simulink model "nimbus"  (R2015b)
settings: Solver=FixedStepDiscrete  SolverMode=SingleTasking  StartTime=0.0  StopTime=sim_stop_time  FixedStep=sim_time_step_size  RelTol=1e-3
PreLoadFcn:
  | nimbus_bus_all;
values from neighbouring files (symbols this model uses):
  sim_time_step_size = 1/100    (= 0.01)    [nimbus_sim_init.m]
undefined symbols (not defined in the file or in its folder): accel, cam_cam1_lander_dcm, cam_cam1_lander_quat, cam_cam1_pos_in_lander, cam_processing_delay_cycles, central_body_flattening, central_body_radius, central_body_rotation_rate, csc_ekf_nonlinear_filter_lib, csc_ekf_nonlinear_filter_new, csc_est_state_est_new, csc_estimation_lib, csc_kfl_kalman_filter_lib, csc_kfl_kalman_filter_new, csc_ldr_flir_lidar, csc_ldr_flir_lidar_lib, csc_rsp_radar_sensor_prep_lib, csc_rsp_radar_sensor_prep_new, csc_sensors_a, csc_sensors_lib_a, csc_sim_simulation, csc_sim_simulation_lib, csc_snp_sensor_prep_lib, csc_snp_sensor_prep_new, csci_fsw, csci_fsw_lib, csci_gsse, csci_gsse_lib, est_time_step, fcv_initializing, ini_alt_wrt_meanrad, ini_epoch_seconds, kfl_lidar_switch_altitude, kfl_use_range_meas, ldr_lander_dcm, ldr_use_meme_flag, pwr_ldr_on_state, q, snp_dtheta_filter_coeffs, snp_dtheta_filter_order, snp_meas_noise_alt, snp_meas_noise_angle, snp_meas_noise_angle_exp, snp_meas_noise_angle_gain, snp_meas_noise_dtheta, snp_meas_noise_dtheta_exp, snp_meas_noise_dtheta_gain, snp_meas_noise_indep, snp_R_lower_limit_alt, snp_R_lower_limit_angle, snp_R_lower_limit_dtheta, snp_rdr_index, snp_rdr_zero_index, snp_zero_index, snp_zero_meas, swm_num_switches, x
undefined symbols (not defined in the file): ldr_position_in_lander
libraries: util_common_lib x23, util_info_lib x13, simulink x8, util_frame_rotation_lib x5, util_quat_lib x5, simulink_extras x4, util_geodesy_lib x2, csu_cfe_cfe_time_lib x2, csu_tlm_telemetry_lib x2, csu_flr_lidar_noise_model_lib x2, csc_act_actuator_manager_lib x1, csc_cmp_command_mode_process_lib x1
(part 1 of 2)
settings Model: SimulationMode=rapid-accelerator  ExtModeTrigDuration=100  Creator=ianmga  LastModifiedBy=Mark Agbayani
settings DataIOCC: LimitDataPoints=off  SaveFormat=Array  SaveOutput=off  SaveTime=off  StateSaveName=tmp_raccel_xout  SignalLoggingName=raw_event_logs
settings OptimizationCC: ExpressionDepthLimit=2147483647  InitFltsAndDblsToZero=on  OptimizeModelRefInitCode=on
settings DebuggingCC: CheckSSInitialOutputMsg=off  UnderspecifiedInitializationDetection=Classic  SolverPrmCheckMsg=warning  InheritedTsInSrcMsg=none  UnderSpecifiedDataTypeMsg=warning  FcnCallInpInsideContextMsg=UseLocalSettings  BusObjectLabelMismatch=error  StateNameClashWarn=warning  StrictBusMsg=WarnOnBusTreatedAsVector
settings HardwareCC: ProdBitPerPointer=32  ProdLargestAtomicFloat=None  ProdIntDivRoundTo=Undefined  ProdEndianess=Unspecified  ProdWordSize=32  ProdHWDeviceType=32-bit Generic  TargetHWDeviceType=32-bit Generic
settings SFSimCC: SimParseCustomCode=off
settings SFSimCC: SimUserIncludeDirs=|
  | sim/fhw/sensors/cameras/kir
  | fsw/est/kcv
  | fsw/est/kfd
  | externals/minopencv/include
settings RTWCC: SystemTargetFile=ert.tlc  GenCodeOnly=on  TemplateMakefile=ert_default_tmf  Description=Embedded Coder  RetainRTWFile=on  RTWUseSimCustomCode=on
settings RTWCC: CustomInclude=|
  | sim/fhw/sensors/cameras/kir
  | fsw/est/kcv
  | fsw/est/kfd
  | externals/minopencv/include
settings CodeAppCC: ForceParamTrailComments=on  IgnoreCustomStorageClasses=off  MaxIdLength=128  SimulinkDataObjDesc=on  SFDataObjDesc=on  MangleLength=10  CustomSymbolStrType=$N$R$M  InsertBlockDesc=on  InternalIdentifier=Classic  ReqsInCode=on
settings ERTTargetCC: GenerateSampleERTMain=on  MultiInstanceERTCode=on  CodeInterfacePackaging=Reusable function  RootIOFormat=Structure reference  ERTCustomFileTemplate=csl_interface.tlc
settings ConfigComp: CovModelRefEnable=Off  CovSFcnEnable=off

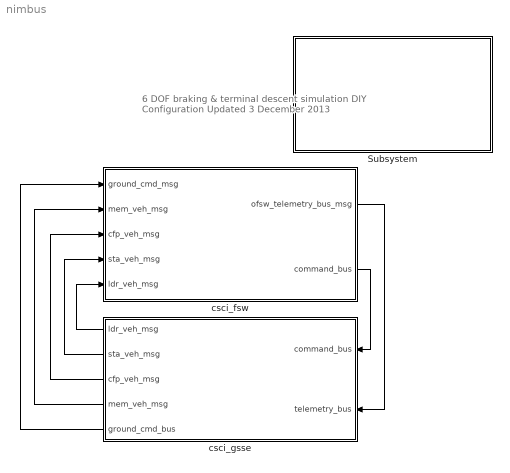
== system nimbus ==
  note: 6 DOF braking & terminal descent simulation
      | DIY Configuration
      |
      | Updated 3 December 2013
  Subsystem : Subsystem
      mask Display: image('nimbus.png')
  csci_fsw : Subsystem  AncestorBlock=csci_fsw_lib/csci_fsw
  csci_gsse : Subsystem  AncestorBlock=csci_gsse_lib/csci_gsse
  wires:
  csci_fsw/2(command_bus) -> csci_gsse/1(command_bus)
  csci_fsw/1(ofsw_telemetry_bus_msg) -> csci_gsse/2(telemetry_bus)
  csci_gsse/1(ldr_veh_msg) -> csci_fsw/5(ldr_veh_msg)
  csci_gsse/2(sta_veh_msg) -> csci_fsw/4(sta_veh_msg)
  csci_gsse/3(cfp_veh_msg) -> csci_fsw/3(cfp_veh_msg)
  csci_gsse/5(ground_cmd_bus) -> csci_fsw/1(ground_cmd_msg)
  csci_gsse/4(mem_veh_msg) -> csci_fsw/2(mem_veh_msg)

== system nimbus/Subsystem ==

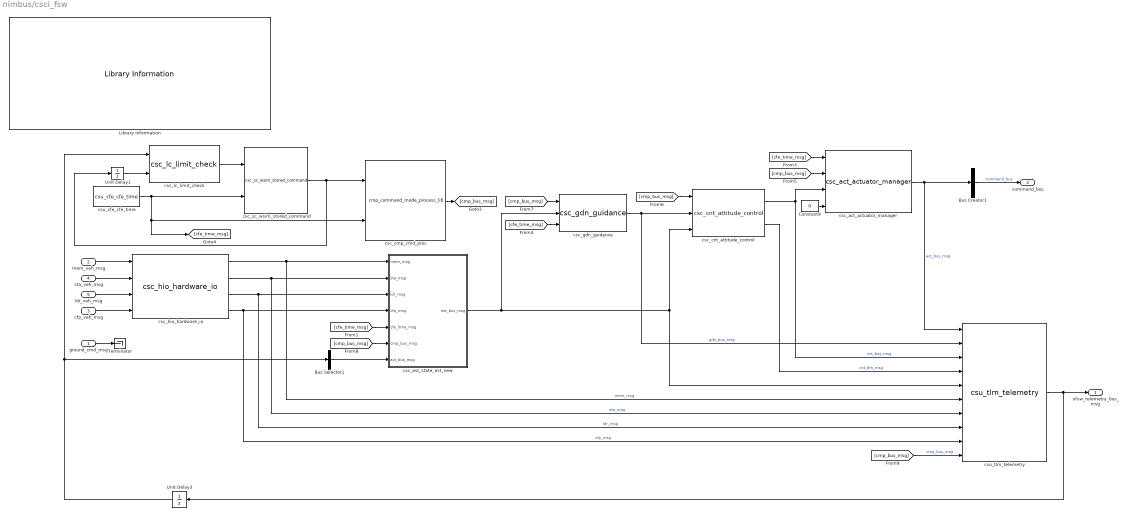
== system nimbus/csci_fsw ==
  ground_cmd_msg : Inport
  mem_veh_msg : Inport  Port=2
  cfp_veh_msg : Inport  Port=3
  sta_veh_msg : Inport  Port=4
  ldr_veh_msg : Inport  Port=5
  Bus Creator1 : BusCreator  Inputs=1
  Bus Selector1 : BusSelector  OutputSignals=act_bus_msg  OutputAsBus=on
  Constant9 : Constant  Value=0  OutDataTypeStr=uint32
  Library Information : util_info_lib/Library Information  owner='NONE'
  Terminator : Terminator
  Unit Delay1 : UnitDelay  SampleTime=-1
  Unit Delay3 : UnitDelay  SampleTime=-1
  csc_act_actuator_manager : csc_act_actuator_manager_lib/csc_act_actuator_manager  Tag=OFSW; MDL_TICK=CNT_BUS_MSG
  csc_cmp_cmd_proc : csc_cmp_command_mode_process_lib/cmp_command_mode_process_lib  Tag=OFSW
  csc_cnt_attitude_control : csc_cnt_attitude_control_lib/csc_cnt_attitude_control  Tag=OFSW; MDL_TICK=GDN_BUS_MSG
  csc_est_state_est_new : Subsystem  Tag=OFSW; MDL_TICK=CMP_BUS_MSG  AncestorBlock=csc_estimation_lib/csc_est_state_est_new  TreatAsAtomicUnit=on  SystemSampleTime=est_time_step
  csc_gdn_guidance : csc_gdn_guidance_lib/csc_gdn_guidance  Tag=OFSW; MDL_TICK=EST_BUS_MSG
  csc_hio_hardware_io : csc_hio_hardware_io_lib/csc_hio_hardware_io
  csc_lc_limit_check : csc_lc_limit_check_lib/csc_lc_limit_check
  csc_sc_wsim_stored_command : csc_sc_wsim_stored_command_lib/csc_sc_wsim_stored_command
  csu_cfe_cfe_time : csu_cfe_cfe_time_lib/csu_cfe_cfe_time  sch_dt=fsw_dt
  csu_tlm_telemetry : csu_tlm_telemetry_lib/csu_tlm_telemetry  num_inputs=10  output_bus_name=ofsw_telemetry_bus_msg
  ofsw_telemetry_bus_msg : Outport
  command_bus : Outport  Port=2
  wires:
  Unit Delay1/1 -> csc_lc_limit_check/2
  Unit Delay3/1 -> csc_lc_limit_check/1, Bus Selector1/1
  csc_lc_limit_check/1 -> csc_sc_wsim_stored_command/1
  [cmp_bus_msg] -> csu_tlm_telemetry/10  "cmp_bus_msg"
  csc_hio_hardware_io/4 -> csc_est_state_est_new/4(cfp_msg), csu_tlm_telemetry/9  "cfp_msg"
  csc_hio_hardware_io/3 -> csc_est_state_est_new/3(ldr_msg), csu_tlm_telemetry/8  "ldr_msg"
  csc_hio_hardware_io/2 -> csc_est_state_est_new/2(sta_msg), csu_tlm_telemetry/7  "sta_msg"
  cfp_veh_msg/1 -> csc_hio_hardware_io/4
  ldr_veh_msg/1 -> csc_hio_hardware_io/3
  sta_veh_msg/1 -> csc_hio_hardware_io/2
  csc_cnt_attitude_control/2 -> csu_tlm_telemetry/4  "cnt_tlm_msg"
  [cmp_bus_msg] -> csc_gdn_guidance/1
  [cmp_bus_msg] -> csc_cnt_attitude_control/1
  [cfe_time_msg] -> csc_est_state_est_new/5(cfe_time_msg)
  csc_cmp_cmd_proc/1 -> [cmp_bus_msg]
  csu_cfe_cfe_time/1 -> [cfe_time_msg], csc_cmp_cmd_proc/2, csc_sc_wsim_stored_command/2
  [cfe_time_msg] -> csc_gdn_guidance/3
  Bus Creator1/1 -> command_bus/1  "command_bus"
  csu_tlm_telemetry/1 -> ofsw_telemetry_bus_msg/1, Unit Delay3/1
  csc_gdn_guidance/1 -> csu_tlm_telemetry/2, csc_cnt_attitude_control/2  "gdn_bus_msg"
  ground_cmd_msg/1 -> Terminator/1
  csc_cnt_attitude_control/1 -> csu_tlm_telemetry/3, csc_act_actuator_manager/3  "cnt_bus_msg"
  csc_est_state_est_new/1(est_bus_msg) -> csc_gdn_guidance/2, csu_tlm_telemetry/5, csc_cnt_attitude_control/3
  csc_sc_wsim_stored_command/1 -> Unit Delay1/1, csc_cmp_cmd_proc/1
  [cmp_bus_msg] -> csc_est_state_est_new/6(cmp_bus_msg)
  Bus Selector1/1 -> csc_est_state_est_new/7(act_bus_msg)
  [cfe_time_msg] -> csc_act_actuator_manager/1
  [cmp_bus_msg] -> csc_act_actuator_manager/2
  csc_act_actuator_manager/1 -> csu_tlm_telemetry/1, Bus Creator1/1  "act_bus_msg"
  Constant9/1 -> csc_act_actuator_manager/4
  mem_veh_msg/1 -> csc_hio_hardware_io/1
  csc_hio_hardware_io/1 -> csc_est_state_est_new/1(mem_msg), csu_tlm_telemetry/6  "mem_msg"

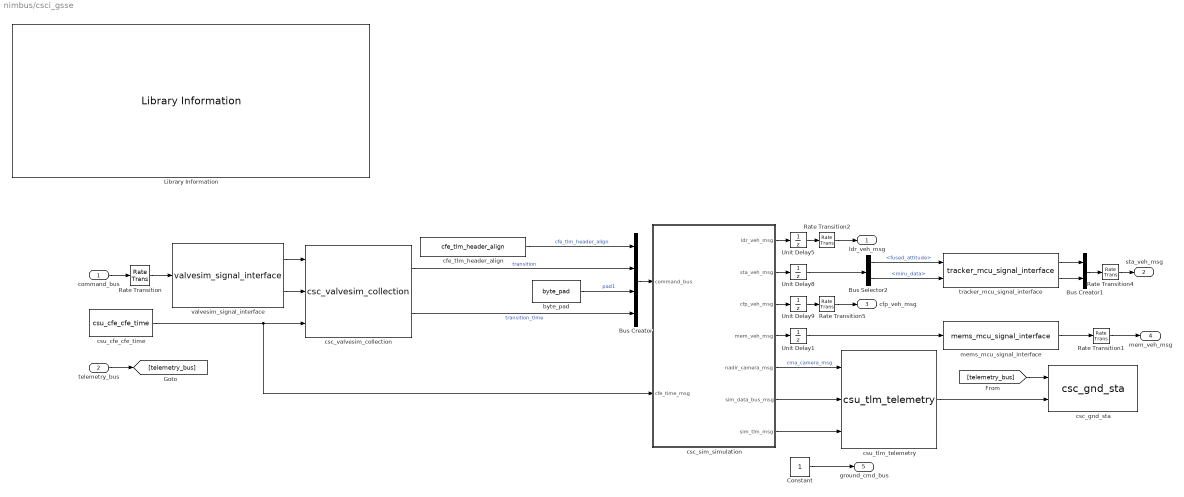
== system nimbus/csci_gsse ==
  command_bus : Inport
  telemetry_bus : Inport  Port=2
  Bus Creator : BusCreator  Inputs=4  OutDataTypeStr=Bus: thr_sim_msg  NonVirtualBus=on
  Bus Selector2 : BusSelector  OutputSignals=fused_attitude,miru_data
  Bus Creator1 : BusCreator  Inputs=2
  Constant : Constant
  Library Information : util_info_lib/Library Information  owner='NONE'
  Rate Transition{,1..2,4..5} (5 alike) : RateTransition  Integrity=off
  Unit Delay{1,5,8..9} (4 alike) : UnitDelay  SampleTime=-1
  byte_pad : util_common_lib/byte_pad  n_bytes=2
  cfe_tlm_header_align : util_common_lib/cfe_tlm_header_align
  csc_gnd_sta : csc_gnd_sta_lib/csc_gnd_sta  dir_name=scenario_data_dir
  csc_sim_simulation : Subsystem  Tag=GSSE; MDL_TICK=THR_SIM_MSG  AncestorBlock=csc_sim_simulation_lib/csc_sim_simulation  TreatAsAtomicUnit=on  SystemSampleTime=sim_time_step_size
  csc_valvesim_collection : csc_valvesim_collection_lib/csc_valvesim_collection  SystemSampleTime=-1
  csu_cfe_cfe_time : csu_cfe_cfe_time_lib/csu_cfe_cfe_time  sch_dt=sim_time_step_size
  csu_tlm_telemetry : csu_tlm_telemetry_lib/csu_tlm_telemetry  num_inputs=3  output_bus_name=sim_telemetry_bus_msg
  mems_mcu_signal_interface : csu_mems_mcu_signal_interface_lib/mems_mcu_signal_interface
  tracker_mcu_signal_interface : csu_tracker_mcu_signal_interface_lib/tracker_mcu_signal_interface
  valvesim_signal_interface : csu_valvesim_signal_interface_lib/valvesim_signal_interface
  ldr_veh_msg : Outport
  sta_veh_msg : Outport  Port=2
  cfp_veh_msg : Outport  Port=3
  mem_veh_msg : Outport  Port=4
  ground_cmd_bus : Outport  Port=5
  wires:
  csu_cfe_cfe_time/1 -> csc_valvesim_collection/3, csc_sim_simulation/2(cfe_time_msg)
  telemetry_bus/1 -> [telemetry_bus]
  csc_sim_simulation/6(sim_data_bus_msg) -> csu_tlm_telemetry/2
  Unit Delay9/1 -> Rate Transition5/1
  Unit Delay5/1 -> Rate Transition2/1
  csc_sim_simulation/1(ldr_veh_msg) -> Unit Delay5/1
  csc_sim_simulation/3(cfp_veh_msg) -> Unit Delay9/1
  Constant/1 -> ground_cmd_bus/1
  command_bus/1 -> Rate Transition/1
  Rate Transition2/1 -> ldr_veh_msg/1
  Rate Transition5/1 -> cfp_veh_msg/1
  csc_sim_simulation/2(sta_veh_msg) -> Unit Delay8/1
  csc_sim_simulation/5(nadir_camera_msg) -> csu_tlm_telemetry/1  "cma_camera_msg"
  csc_sim_simulation/7(sim_tlm_msg) -> csu_tlm_telemetry/3
  csu_tlm_telemetry/1 -> csc_gnd_sta/2
  [telemetry_bus] -> csc_gnd_sta/1
  Rate Transition/1 -> valvesim_signal_interface/1
  valvesim_signal_interface/1 -> csc_valvesim_collection/1
  csc_valvesim_collection/1 -> Bus Creator/2  "transition"
  csc_valvesim_collection/2 -> Bus Creator/4  "transition_time"
  Bus Creator/1 -> csc_sim_simulation/1(command_bus)
  byte_pad/1 -> Bus Creator/3  "pad1"
  cfe_tlm_header_align/1 -> Bus Creator/1  "cfe_tlm_header_align"
  valvesim_signal_interface/2 -> csc_valvesim_collection/2
  Bus Selector2/1 -> tracker_mcu_signal_interface/1  "<fused_attitude>"
  Bus Selector2/2 -> tracker_mcu_signal_interface/2  "<miru_data>"
  Unit Delay8/1 -> Bus Selector2/1
  tracker_mcu_signal_interface/1 -> Bus Creator1/1
  tracker_mcu_signal_interface/2 -> Bus Creator1/2
  Bus Creator1/1 -> Rate Transition4/1
  Rate Transition4/1 -> sta_veh_msg/1
  csc_sim_simulation/4(mem_veh_msg) -> Unit Delay1/1
  Unit Delay1/1 -> mems_mcu_signal_interface/1
  mems_mcu_signal_interface/1 -> Rate Transition1/1
  Rate Transition1/1 -> mem_veh_msg/1

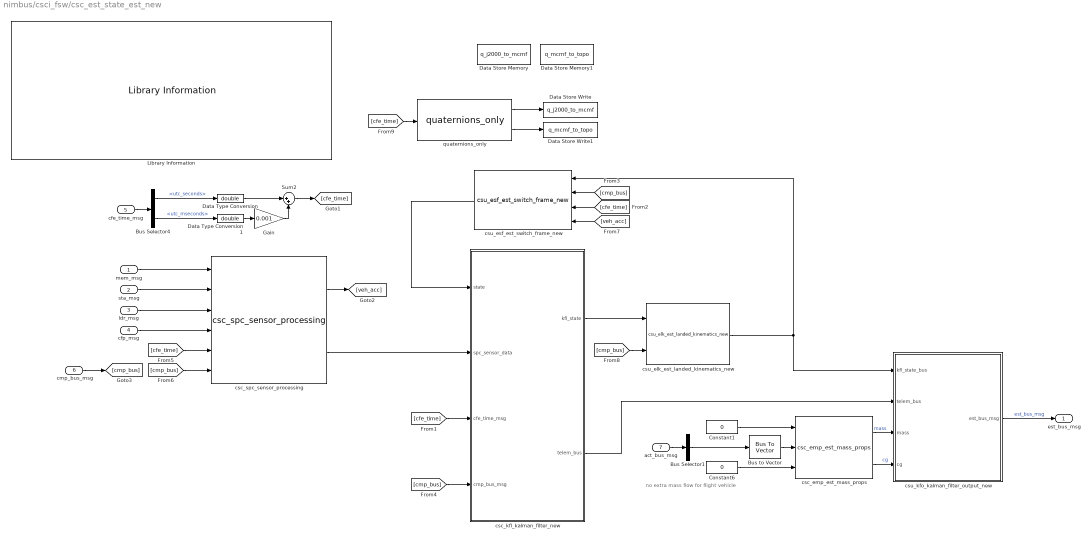
== system nimbus/csci_fsw/csc_est_state_est_new ==
  note: no extra mass flow for flight vehicle
  mem_msg : Inport  OutDataTypeStr=Bus: mem_msg
  sta_msg : Inport  Port=2  OutDataTypeStr=Bus: sta_msg
  ldr_msg : Inport  Port=3  OutDataTypeStr=Bus: ldr_msg
  cfp_msg : Inport  Port=4  OutDataTypeStr=Bus: cfp_msg
  cfe_time_msg : Inport  Port=5  OutDataTypeStr=Bus: cfe_time_msg
  cmp_bus_msg : Inport  Port=6  OutDataTypeStr=Bus: cmp_bus_msg
  act_bus_msg : Inport  Port=7  OutDataTypeStr=Bus: act_bus_msg
  Bus Selector1 : BusSelector  OutputSignals=coarse1_time,coarse2_time,coarse3_time,coarse4_time,coarse5_time,coarse6_time,coarse7_time,coarse8_time,coarse9_time,coarse10_time,coarse11_time,coarse12_time,fine1_time,fine2_time,fine3_time,fine4_time,fine5_time,fine6_time,fine7_time,fine8_time,fine9_time,fine10_time,fine11_time,fine12_time,main_thruster_cmd,main_biprop_monoprop  OutputAsBus=on
  Bus Selector4 : BusSelector  OutputSignals=utc_seconds,utc_mseconds
  Bus to Vector : BusToVector
  Constant1 : Constant  Value=0
  Constant6 : Constant  Value=0
  Data Store Memory : DataStoreMemory  DataStoreName=q_j2000_to_mcmf  ReadBeforeWriteMsg=warning  WriteAfterWriteMsg=warning  WriteAfterReadMsg=warning  InitialValue=[0 0 0 1]  OutDataTypeStr=double
  Data Store Memory1 : DataStoreMemory  DataStoreName=q_mcmf_to_topo  ReadBeforeWriteMsg=warning  WriteAfterWriteMsg=warning  WriteAfterReadMsg=warning  InitialValue=[0 0 0 1]  OutDataTypeStr=double
  Data Store Write : DataStoreWrite  DataStoreName=q_j2000_to_mcmf
  Data Store Write1 : DataStoreWrite  DataStoreName=q_mcmf_to_topo
  Data Type Conversion : DataTypeConversion  OutDataTypeStr=double
  Data Type Conversion1 : DataTypeConversion  OutDataTypeStr=double
  Gain : Gain  Gain=0.001
  Library Information : util_info_lib/Library Information  owner='NONE'
  Sum2 : Sum  Inputs=|++
  csc_emp_est_mass_props : csc_emp_est_mass_props_lib/csc_emp_est_mass_props
  csc_kfl_kalman_filter_new : Subsystem  AncestorBlock=csc_kfl_kalman_filter_lib/csc_kfl_kalman_filter_new
  csc_spc_sensor_processing : csc_spc_sensor_processing_lib/csc_spc_sensor_processing
  csu_elk_est_landed_kinematics_new : csu_elk_est_landed_kinematics_lib/csu_elk_est_landed_kinematics_new
  csu_esf_est_switch_frame_new : csu_esf_est_switch_frame_lib/csu_esf_est_switch_frame_new
  csu_kfo_kalman_filter_output_new : Subsystem
  quaternions_only : util_frame_rotation_lib/quaternions_only  SystemSampleTime=-1
  est_bus_msg : Outport  OutDataTypeStr=Bus: est_bus_msg
  wires:
  csc_emp_est_mass_props/1 -> csu_kfo_kalman_filter_output_new/3(mass)  "mass"
  csc_emp_est_mass_props/2 -> csu_kfo_kalman_filter_output_new/4(cg)  "cg"
  Constant6/1 -> csc_emp_est_mass_props/3
  cfp_msg/1 -> csc_spc_sensor_processing/4
  csu_kfo_kalman_filter_output_new/1(est_bus_msg) -> est_bus_msg/1  "est_bus_msg"
  csu_esf_est_switch_frame_new/1 -> csc_kfl_kalman_filter_new/1(state)
  cmp_bus_msg/1 -> [cmp_bus]
  [cfe_time] -> csu_esf_est_switch_frame_new/3
  [cmp_bus] -> csu_esf_est_switch_frame_new/2
  [cfe_time] -> csc_kfl_kalman_filter_new/3(cfe_time_msg)
  [cmp_bus] -> csc_kfl_kalman_filter_new/4(cmp_bus_msg)
  sta_msg/1 -> csc_spc_sensor_processing/2
  ldr_msg/1 -> csc_spc_sensor_processing/3
  [cfe_time] -> csc_spc_sensor_processing/5
  [cmp_bus] -> csc_spc_sensor_processing/6
  csc_spc_sensor_processing/2 -> csc_kfl_kalman_filter_new/2(spc_sensor_data)
  csc_kfl_kalman_filter_new/1(kfl_state) -> csu_elk_est_landed_kinematics_new/1
  csu_elk_est_landed_kinematics_new/1 -> csu_esf_est_switch_frame_new/1, csu_kfo_kalman_filter_output_new/1(kfl_state_bus)
  [cmp_bus] -> csu_elk_est_landed_kinematics_new/2
  [veh_acc] -> csu_esf_est_switch_frame_new/4
  Gain/1 -> Sum2/2
  Data Type Conversion1/1 -> Gain/1
  Data Type Conversion/1 -> Sum2/1
  Bus Selector4/1 -> Data Type Conversion/1  "<utc_seconds>"
  Bus Selector4/2 -> Data Type Conversion1/1  "<utc_mseconds>"
  Sum2/1 -> [cfe_time]
  cfe_time_msg/1 -> Bus Selector4/1
  csc_kfl_kalman_filter_new/2(telem_bus) -> csu_kfo_kalman_filter_output_new/2(telem_bus)
  csc_spc_sensor_processing/1 -> [veh_acc]
  [cfe_time] -> quaternions_only/1
  quaternions_only/1 -> Data Store Write/1
  quaternions_only/2 -> Data Store Write1/1
  mem_msg/1 -> csc_spc_sensor_processing/1
  Constant1/1 -> csc_emp_est_mass_props/1
  act_bus_msg/1 -> Bus Selector1/1
  Bus to Vector/1 -> csc_emp_est_mass_props/2
  Bus Selector1/1 -> Bus to Vector/1

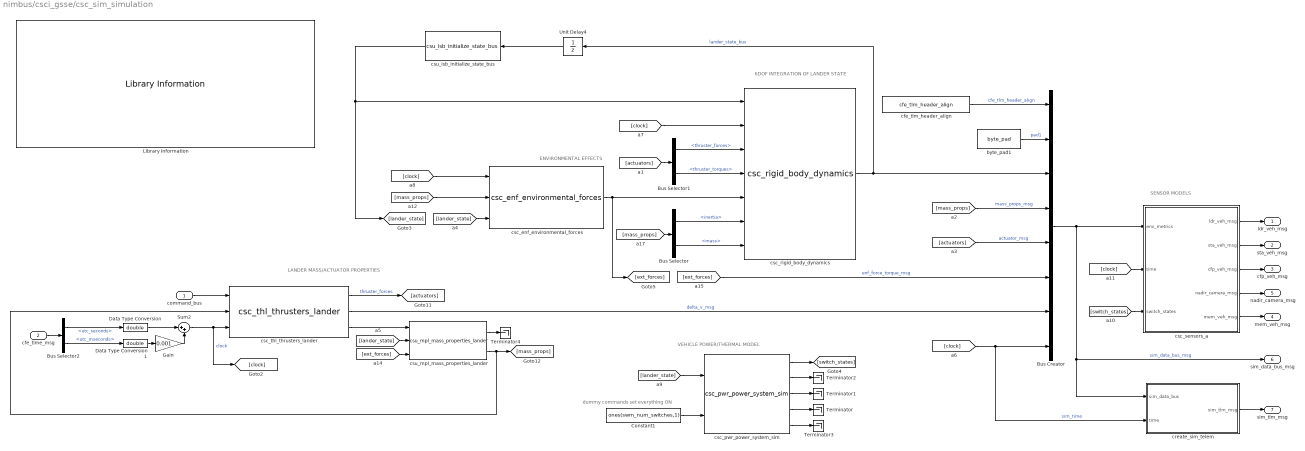
== system nimbus/csci_gsse/csc_sim_simulation ==
  note: dummy commands set everything ON
  note: VEHICLE POWER/THERMAL MODEL
  note: SENSOR MODELS
  note: ENVIRONMENTAL EFFECTS
  note: 6DOF INTEGRATION OF LANDER STATE
  note: LANDER MASS/ACTUATOR PROPERTIES
  command_bus : Inport
  cfe_time_msg : Inport  Port=2  OutDataTypeStr=Bus: cfe_time_msg
  Bus Creator : BusCreator  Inputs=8  OutDataTypeStr=Bus: sim_data_bus_msg  NonVirtualBus=on
  Bus Selector : BusSelector  OutputSignals=inertia,mass
  Bus Selector1 : BusSelector  OutputSignals=thruster_forces,thruster_torques
  Bus Selector2 : BusSelector  OutputSignals=utc_seconds,utc_mseconds
  Constant1 : Constant  Value=ones(swm_num_switches,1)  OutDataTypeStr=double
  Data Type Conversion : DataTypeConversion  OutDataTypeStr=double
  Data Type Conversion1 : DataTypeConversion  OutDataTypeStr=double
  Gain : Gain  Gain=0.001
  Library Information : util_info_lib/Library Information  owner='NONE'
  Sum2 : Sum  Inputs=|++
  Terminator{,1..4} (5 alike) : Terminator
  Unit Delay4 : UnitDelay  SampleTime=-1
  byte_pad1 : util_common_lib/byte_pad  n_bytes=4
  cfe_tlm_header_align : util_common_lib/cfe_tlm_header_align
  create_sim_telem : Subsystem
  csc_enf_environmental_forces : csc_enf_environmental_forces_lib/csc_enf_environmental_forces
  csc_pwr_power_system_sim : csc_pwr_power_system_sim_lib/csc_pwr_power_system_sim
  csc_rigid_body_dynamics : csc_rigid_body_dynamics_lib/csc_rigid_body_dynamics
  csc_sensors_a : Subsystem  AncestorBlock=csc_sensors_lib_a/csc_sensors_a
  csc_thl_thrusters_lander : csc_thl_thrusters_lander_lib/csc_thl_thrusters_lander
  csu_isb_initialize_state_bus : csu_isb_initialize_state_bus_lib/csu_isb_initialize_state_bus
  csu_mpl_mass_properties_lander : csu_mpl_mass_properties_lander_lib/csu_mpl_mass_properties_lander
  ldr_veh_msg : Outport
  sta_veh_msg : Outport  Port=2
  cfp_veh_msg : Outport  Port=3
  mem_veh_msg : Outport  Port=4
  nadir_camera_msg : Outport  Port=5
  sim_data_bus_msg : Outport  Port=6
  sim_tlm_msg : Outport  Port=7
  wires:
  [ext_forces] -> Bus Creator/6  "enf_force_torque_msg"
  csc_enf_environmental_forces/1 -> csc_rigid_body_dynamics/5, [ext_forces]
  [ext_forces] -> csu_mpl_mass_properties_lander/3
  [lander_state] -> csu_mpl_mass_properties_lander/2
  csu_mpl_mass_properties_lander/1 -> Terminator4/1
  csc_pwr_power_system_sim/5 -> Terminator3/1
  csc_sensors_a/5(mem_veh_msg) -> mem_veh_msg/1
  Constant1/1 -> csc_pwr_power_system_sim/2
  [switch_states] -> csc_sensors_a/3(switch_states)
  [clock] -> csc_sensors_a/2(time)
  [lander_state] -> csc_pwr_power_system_sim/1
  [lander_state] -> csc_enf_environmental_forces/3
  csc_pwr_power_system_sim/1 -> [switch_states]
  csc_pwr_power_system_sim/2 -> Terminator2/1
  csc_pwr_power_system_sim/3 -> Terminator1/1
  csc_pwr_power_system_sim/4 -> Terminator/1
  [actuators] -> Bus Selector1/1
  csu_isb_initialize_state_bus/1 -> [lander_state], csc_rigid_body_dynamics/1
  Unit Delay4/1 -> csu_isb_initialize_state_bus/1
  Bus Selector1/2 -> csc_rigid_body_dynamics/4  "<thruster_torques>"
  Bus Selector1/1 -> csc_rigid_body_dynamics/3  "<thruster_forces>"
  Bus Selector/1 -> csc_rigid_body_dynamics/6  "<inertia>"
  Bus Selector/2 -> csc_rigid_body_dynamics/7  "<mass>"
  [mass_props] -> Bus Selector/1
  [clock] -> csc_rigid_body_dynamics/2
  cfe_tlm_header_align/1 -> Bus Creator/1  "cfe_tlm_header_align"
  [mass_props] -> csc_enf_environmental_forces/2
  [clock] -> csc_enf_environmental_forces/1
  csc_thl_thrusters_lander/2 -> Bus Creator/7  "delta_v_msg"
  csc_thl_thrusters_lander/1 -> [actuators]  "thruster_forces"
  csc_thl_thrusters_lander/3 -> csu_mpl_mass_properties_lander/1
  csc_sensors_a/1(ldr_veh_msg) -> ldr_veh_msg/1
  csc_sensors_a/2(sta_veh_msg) -> sta_veh_msg/1
  csu_mpl_mass_properties_lander/2 -> [mass_props], csc_thl_thrusters_lander/2
  [mass_props] -> Bus Creator/4  "mass_props_msg"
  [actuators] -> Bus Creator/5  "actuator_msg"
  command_bus/1 -> csc_thl_thrusters_lander/1
  csc_sensors_a/4(nadir_camera_msg) -> nadir_camera_msg/1
  csc_sensors_a/3(cfp_veh_msg) -> cfp_veh_msg/1
  csc_rigid_body_dynamics/1 -> Unit Delay4/1, Bus Creator/3  "lander_state_bus"
  Bus Creator/1 -> csc_sensors_a/1(env_metrics), sim_data_bus_msg/1, create_sim_telem/1(sim_data_bus)  "sim_data_bus_msg"
  create_sim_telem/1(sim_tlm_msg) -> sim_tlm_msg/1
  [clock] -> Bus Creator/8, create_sim_telem/2(time)  "sim_time"
  Sum2/1 -> [clock], csc_thl_thrusters_lander/3  "clock"
  byte_pad1/1 -> Bus Creator/2  "pad1"
  Bus Selector2/1 -> Data Type Conversion/1  "<utc_seconds>"
  Gain/1 -> Sum2/2
  Data Type Conversion1/1 -> Gain/1
  Data Type Conversion/1 -> Sum2/1
  Bus Selector2/2 -> Data Type Conversion1/1  "<utc_mseconds>"
  cfe_time_msg/1 -> Bus Selector2/1

== system nimbus/csci_fsw/csc_est_state_est_new/csc_kfl_kalman_filter_new ==
  state : Inport
  spc_sensor_data : Inport  Port=2
  cfe_time_msg : Inport  Port=3
  cmp_bus_msg : Inport  Port=4
  Bus Selector5 : BusSelector  OutputSignals=mem_msg,sta_msg,ldr_msg,feature_data
  Library Information : util_info_lib/Library Information  owner='NONE'
  csc_ekf_nonlinear_filter_new : Subsystem  AncestorBlock=csc_ekf_nonlinear_filter_lib/csc_ekf_nonlinear_filter_new
  csc_snp_sensor_prep_new : Subsystem  AncestorBlock=csc_snp_sensor_prep_lib/csc_snp_sensor_prep_new
  kfl_state : Outport
  telem_bus : Outport  Port=2
  wires:
  cmp_bus_msg/1 -> csc_ekf_nonlinear_filter_new/4(cmp_bus_msg), csc_snp_sensor_prep_new/7(cmp_bus)
  csc_ekf_nonlinear_filter_new/1(new_state_bus) -> kfl_state/1
  state/1 -> csc_snp_sensor_prep_new/6(state_in), csc_ekf_nonlinear_filter_new/2(old_state_bus)
  cfe_time_msg/1 -> csc_snp_sensor_prep_new/5(cfe_time_msg), csc_ekf_nonlinear_filter_new/3(cfe_time_msg)
  csc_snp_sensor_prep_new/1(sensor_data_bus) -> csc_ekf_nonlinear_filter_new/1(sensor_bus)
  spc_sensor_data/1 -> Bus Selector5/1
  Bus Selector5/3 -> csc_snp_sensor_prep_new/3(radar_data)  "<ldr_msg>"
  Bus Selector5/4 -> csc_snp_sensor_prep_new/4(feature_data)  "<feature_data>"
  Bus Selector5/1 -> csc_snp_sensor_prep_new/1(mems_data)  "<mem_msg>"
  csc_ekf_nonlinear_filter_new/2(telem_bus) -> telem_bus/1
  Bus Selector5/2 -> csc_snp_sensor_prep_new/2(sta_data)  "<sta_msg>"

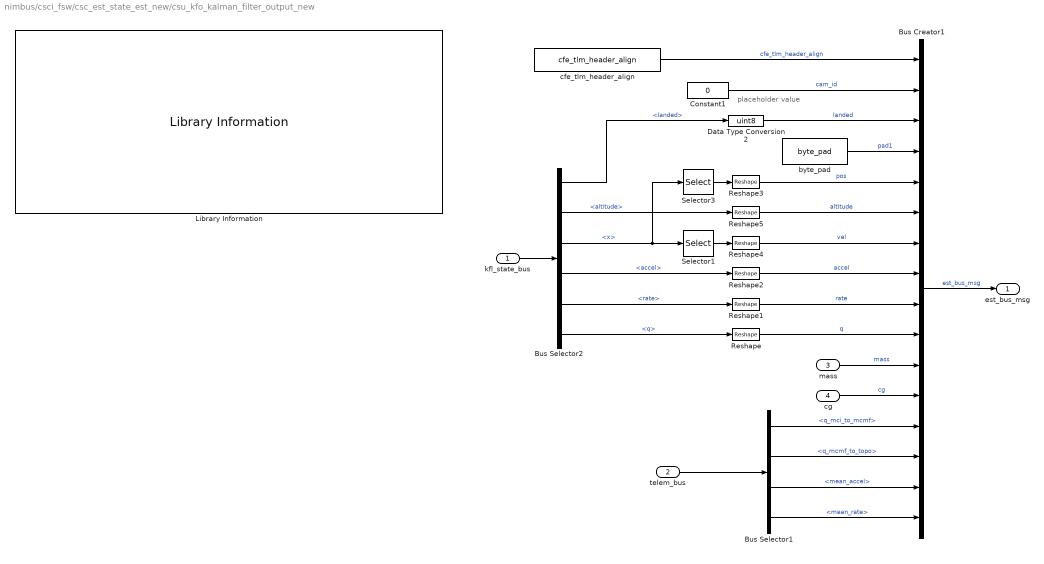
== system nimbus/csci_fsw/csc_est_state_est_new/csu_kfo_kalman_filter_output_new ==
  note: placeholder value
  kfl_state_bus : Inport
  telem_bus : Inport  Port=2
  mass : Inport  Port=3
  cg : Inport  Port=4
  Bus Creator1 : BusCreator  Inputs=16  OutDataTypeStr=Bus: est_bus_msg  NonVirtualBus=on
  Bus Selector1 : BusSelector  OutputSignals=q_mci_to_mcmf,q_mcmf_to_topo,mean_accel,mean_rate
  Bus Selector2 : BusSelector  OutputSignals=landed,altitude,x,accel,rate,q
  Constant1 : Constant  Value=0  OutDataTypeStr=uint8
  Data Type Conversion2 : DataTypeConversion  OutDataTypeStr=uint8
  Library Information : util_info_lib/Library Information  owner='escrane'
  Reshape{,1..5} (6 alike) : Reshape
  Selector1 : Selector  InputPortWidth=kfl_n_state  IndexOptions=Index vector (dialog)  Indices=kfl_vel_index  OutputSizes=1
  Selector3 : Selector  InputPortWidth=kfl_n_state  IndexOptions=Index vector (dialog)  Indices=kfl_pos_index  OutputSizes=1
  byte_pad : util_common_lib/byte_pad  n_bytes=2
  cfe_tlm_header_align : util_common_lib/cfe_tlm_header_align
  est_bus_msg : Outport
  wires:
  Bus Selector2/2 -> Reshape5/1  "<altitude>"
  Data Type Conversion2/1 -> Bus Creator1/3  "landed"
  Selector3/1 -> Reshape3/1
  Reshape3/1 -> Bus Creator1/5  "pos"
  Reshape4/1 -> Bus Creator1/7  "vel"
  Reshape1/1 -> Bus Creator1/9  "rate"
  Reshape/1 -> Bus Creator1/10  "q"
  Bus Selector2/3 -> Selector3/1, Selector1/1  "<x>"
  Selector1/1 -> Reshape4/1
  Bus Selector2/4 -> Reshape2/1  "<accel>"
  Bus Selector2/5 -> Reshape1/1  "<rate>"
  Bus Selector2/6 -> Reshape/1  "<q>"
  Bus Creator1/1 -> est_bus_msg/1  "est_bus_msg"
  Reshape2/1 -> Bus Creator1/8  "accel"
  Constant1/1 -> Bus Creator1/2  "cam_id"
  byte_pad/1 -> Bus Creator1/4  "pad1"
  Bus Selector2/1 -> Data Type Conversion2/1  "<landed>"
  cfe_tlm_header_align/1 -> Bus Creator1/1  "cfe_tlm_header_align"
  kfl_state_bus/1 -> Bus Selector2/1
  mass/1 -> Bus Creator1/11  "mass"
  cg/1 -> Bus Creator1/12  "cg"
  telem_bus/1 -> Bus Selector1/1
  Bus Selector1/2 -> Bus Creator1/14  "<q_mcmf_to_topo>"
  Bus Selector1/1 -> Bus Creator1/13  "<q_mci_to_mcmf>"
  Bus Selector1/3 -> Bus Creator1/15  "<mean_accel>"
  Bus Selector1/4 -> Bus Creator1/16  "<mean_rate>"
  Reshape5/1 -> Bus Creator1/6  "altitude"

== system nimbus/csci_gsse/csc_sim_simulation/create_sim_telem ==
  sim_data_bus : Inport
  time : Inport  Port=2
  Bus Creator : BusCreator  Inputs=13  OutDataTypeStr=Bus: sim_tlm_msg  NonVirtualBus=on
  Bus Selector2 : BusSelector  OutputSignals=lander_state_bus.rtk_pos_eci,lander_state_bus.rtk_vel_eci,lander_state_bus.rrk_q_body_from_eci,lander_state_bus.rtd_acc_body_in_eci,lander_state_bus.spacecraft_landed_flag,lander_state_bus.rrk_rate_body_eci_body,mass_props_msg.mass
  Constant1 : Constant  Value=ini_alt_wrt_meanrad  OutDataTypeStr=double
  Constant2 : Constant  Value=ini_epoch_seconds  OutDataTypeStr=double
  Constant4 : Constant  Value=0
  Gain : Gain
  Gain1 : Gain
  Sum1 : Sum  Inputs=|+-
  Sum2 : Sum  Inputs=|+-
  Terminator2 : Terminator
  Terminator3 : Terminator
  byte_pad1 : util_common_lib/byte_pad  n_bytes=4
  cbi_to_lla : util_frame_rotation_lib/cbi_to_lla  a=central_body_radius  b=central_body_radius*(1-central_body_flattening)  omega=central_body_rotation_rate(3)
  cfe_tlm_header_align : util_common_lib/cfe_tlm_header_align
  kinematic_telemetry_conversion : telem_conversion_lib/kinematic_telemetry_conversion
  time1 : InportShadow  Port=2
  sim_tlm_msg : Outport
  wires:
  byte_pad1/1 -> Bus Creator/2  "pad1"
  kinematic_telemetry_conversion/3 -> Terminator3/1
  kinematic_telemetry_conversion/2 -> Terminator2/1
  Bus Creator/1 -> sim_tlm_msg/1  "sim_tlm_msg"
  kinematic_telemetry_conversion/8 -> Bus Creator/7  "acc_topo"
  kinematic_telemetry_conversion/7 -> Bus Creator/6  "euler_zyx"
  kinematic_telemetry_conversion/6 -> Bus Creator/5  "q_topo_to_body"
  kinematic_telemetry_conversion/5 -> Bus Creator/4  "vel_topo"
  sim_data_bus/1 -> Bus Selector2/1
  time/1 -> kinematic_telemetry_conversion/1
  Bus Selector2/1 -> kinematic_telemetry_conversion/2  "<rtk_pos_eci>"
  Bus Selector2/2 -> kinematic_telemetry_conversion/3  "<rtk_vel_eci>"
  Bus Selector2/3 -> kinematic_telemetry_conversion/4  "<rrk_q_body_from_eci>"
  Bus Selector2/4 -> kinematic_telemetry_conversion/5  "<rtd_acc_body_in_eci>"
  Bus Selector2/6 -> Gain/1  "<rrk_rate_body_eci_body>"
  Gain/1 -> Bus Creator/8  "rate_body"
  Bus Selector2/7 -> Gain1/1  "<mass>"
  Gain1/1 -> Bus Creator/9  "mass"
  kinematic_telemetry_conversion/4 -> Bus Creator/3  "pos_topo"
  cfe_tlm_header_align/1 -> Bus Creator/1  "cfe_tlm_header_align"
  Bus Selector2/5 -> kinematic_telemetry_conversion/6  "<spacecraft_landed_flag>"
  cbi_to_lla/2 -> Bus Creator/11  "detic_latitude"
  cbi_to_lla/1 -> Bus Creator/10  "centric_latitude"
  cbi_to_lla/3 -> Bus Creator/12  "longitude"
  Sum2/1 -> Bus Creator/13  "altitude"
  Constant4/1 -> cbi_to_lla/2
  Sum1/1 -> cbi_to_lla/1
  time1/1 -> Sum1/1
  Constant2/1 -> Sum1/2
  [pos_mcmf] -> cbi_to_lla/3
  kinematic_telemetry_conversion/1 -> [pos_mcmf]
  cbi_to_lla/4 -> Sum2/1
  Constant1/1 -> Sum2/2

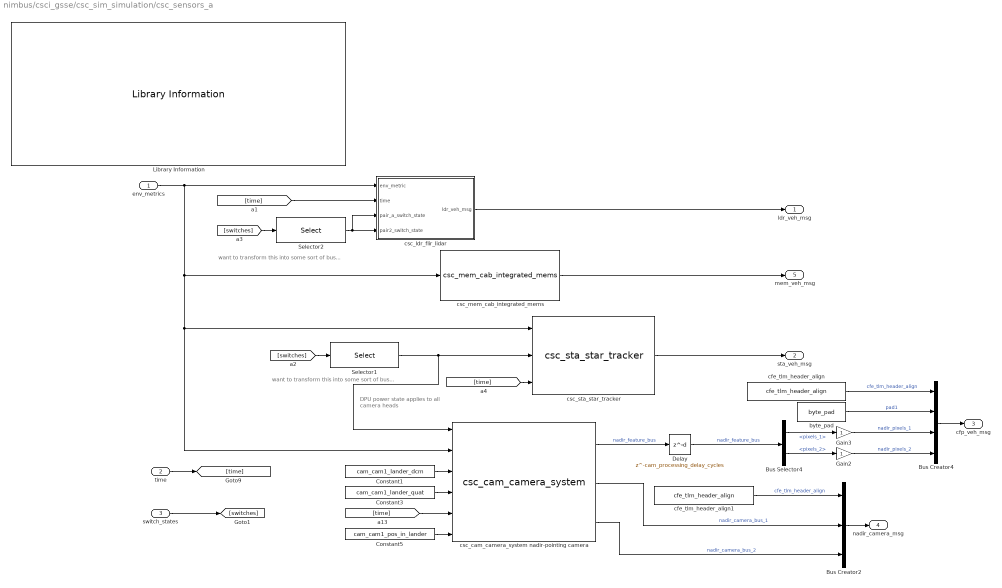
== system nimbus/csci_gsse/csc_sim_simulation/csc_sensors_a ==
  note: DPU power state applies
      | to all camera heads
  note: want to transform this into some sort of bus...
  note: want to transform this into some sort of bus...
  env_metrics : Inport
  time : Inport  Port=2
  switch_states : Inport  Port=3
  Bus Creator2 : BusCreator  Inputs=3  NonVirtualBus=on
  Bus Creator4 : BusCreator  Inputs=4  OutDataTypeStr=Bus: cfp_veh_msg  NonVirtualBus=on
  Bus Selector4 : BusSelector  OutputSignals=pixels_1,pixels_2
  Constant1 : Constant  Value=cam_cam1_lander_dcm
  Constant3 : Constant  Value=cam_cam1_lander_quat
  Constant5 : Constant  Value=cam_cam1_pos_in_lander
  Delay : Delay  DelayLength=cam_processing_delay_cycles
  Gain2 : Gain
  Gain3 : Gain
  Library Information : util_info_lib/Library Information  owner='NONE'
  Selector1 : Selector  InputPortWidth=swm_num_switches  IndexOptions=Index vector (dialog)  Indices=1  OutputSizes=1
  Selector2 : Selector  InputPortWidth=swm_num_switches  IndexOptions=Index vector (dialog)  Indices=2  OutputSizes=1
  byte_pad : util_common_lib/byte_pad  n_bytes=4
  cfe_tlm_header_align : util_common_lib/cfe_tlm_header_align
  cfe_tlm_header_align1 : util_common_lib/cfe_tlm_header_align
  csc_cam_camera_system nadir-pointing camera : csc_cam_camera_system_lib/csc_cam_camera_system
  csc_ldr_flir_lidar : Subsystem  AncestorBlock=csc_ldr_flir_lidar_lib/csc_ldr_flir_lidar  SystemSampleTime=0.1
  csc_mem_cab_integrated_mems : csc_mem_cab_integrated_mems_lib/csc_mem_cab_integrated_mems
  csc_sta_star_tracker : csc_sta_star_tracker_lib/csc_sta_star_tracker
  ldr_veh_msg : Outport
  sta_veh_msg : Outport  Port=2
  cfp_veh_msg : Outport  Port=3
  nadir_camera_msg : Outport  Port=4
  mem_veh_msg : Outport  Port=5
  wires:
  Gain2/1 -> Bus Creator4/4  "nadir_pixels_2"
  Gain3/1 -> Bus Creator4/3  "nadir_pixels_1"
  Bus Selector4/1 -> Gain3/1  "<pixels_1>"
  Delay/1 -> Bus Selector4/1  "nadir_feature_bus"
  Bus Creator4/1 -> cfp_veh_msg/1
  csc_cam_camera_system nadir-pointing camera/2 -> Bus Creator2/2  "nadir_camera_bus_1"
  csc_cam_camera_system nadir-pointing camera/1 -> Delay/1  "nadir_feature_bus"
  Constant1/1 -> csc_cam_camera_system nadir-pointing camera/3
  env_metrics/1 -> csc_ldr_flir_lidar/1(env_metric), csc_mem_cab_integrated_mems/1, csc_sta_star_tracker/1, csc_cam_camera_system nadir-pointing camera/2
  csc_sta_star_tracker/1 -> sta_veh_msg/1
  csc_ldr_flir_lidar/1(ldr_veh_msg) -> ldr_veh_msg/1
  Bus Creator2/1 -> nadir_camera_msg/1
  Constant3/1 -> csc_cam_camera_system nadir-pointing camera/4
  time/1 -> [time]
  [time] -> csc_cam_camera_system nadir-pointing camera/5
  [time] -> csc_ldr_flir_lidar/2(time)
  Constant5/1 -> csc_cam_camera_system nadir-pointing camera/6
  Bus Selector4/2 -> Gain2/1  "<pixels_2>"
  byte_pad/1 -> Bus Creator4/2  "pad1"
  cfe_tlm_header_align/1 -> Bus Creator4/1  "cfe_tlm_header_align"
  cfe_tlm_header_align1/1 -> Bus Creator2/1  "cfe_tlm_header_align"
  csc_cam_camera_system nadir-pointing camera/3 -> Bus Creator2/3  "nadir_camera_bus_2"
  Selector1/1 -> csc_sta_star_tracker/2, csc_cam_camera_system nadir-pointing camera/1
  switch_states/1 -> [switches]
  [switches] -> Selector1/1
  [switches] -> Selector2/1
  Selector2/1 -> csc_ldr_flir_lidar/3(pair_a_switch_state), csc_ldr_flir_lidar/4(pair2_switch_state)
  [time] -> csc_sta_star_tracker/3
  csc_mem_cab_integrated_mems/1 -> mem_veh_msg/1

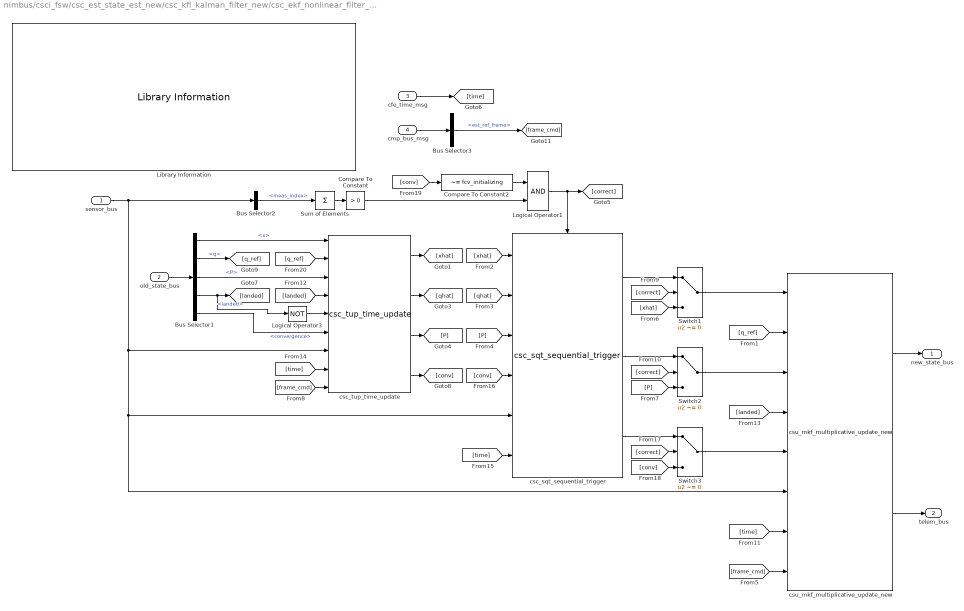
== system nimbus/csci_fsw/csc_est_state_est_new/csc_kfl_kalman_filter_new/csc_ekf_nonlinear_filter_new ==
  sensor_bus : Inport
  old_state_bus : Inport  Port=2
  cfe_time_msg : Inport  Port=3
  cmp_bus_msg : Inport  Port=4
  Bus Selector1 : BusSelector  OutputSignals=x,q,P,landed,convergence
  Bus Selector2 : BusSelector  OutputSignals=meas_index
  Bus Selector3 : BusSelector  OutputSignals=est_ref_frame
  Compare To Constant : simulink/Logic and Bit Operations/Compare To Constant  relop=>  const=0  OutDataTypeStr=uint8  ZeroCross=off
  Compare To Constant2 : simulink/Logic and Bit Operations/Compare To Constant  relop=~=  const=fcv_initializing  OutDataTypeStr=boolean
  Library Information : util_info_lib/Library Information  owner='NONE'
  Logical Operator1 : Logic  AllPortsSameDT=off  OutDataTypeStr=boolean
  Logical Operator3 : Logic  Operator=NOT  AllPortsSameDT=off  OutDataTypeStr=boolean
  Sum of Elements : Sum  Inputs=+
  Switch1 : Switch  Criteria=u2 ~= 0  Threshold=0.5  InputSameDT=on
  Switch2 : Switch  Criteria=u2 ~= 0  Threshold=0.5  InputSameDT=on
  Switch3 : Switch  Criteria=u2 ~= 0  Threshold=0.5  InputSameDT=on
  csc_sqt_sequential_trigger : csc_sqt_sequential_trigger_lib/csc_sqt_sequential_trigger
  csc_tup_time_update : csc_tup_time_update_lib/csc_tup_time_update
  csu_mkf_multiplicative_update_new : csu_mkf_multiplicative_update_lib/csu_mkf_multiplicative_update_new
  new_state_bus : Outport
  telem_bus : Outport  Port=2
  wires:
  Switch2/1 -> csu_mkf_multiplicative_update_new/3
  Switch3/1 -> csu_mkf_multiplicative_update_new/5
  Logical Operator3/1 -> csc_tup_time_update/5
  Compare To Constant/1 -> Logical Operator1/2
  Compare To Constant2/1 -> Logical Operator1/1
  [conv] -> Compare To Constant2/1
  Logical Operator1/1 -> csc_sqt_sequential_trigger/Enable, [correct]
  csc_sqt_sequential_trigger/3 -> Switch3/1
  [conv] -> Switch3/3
  [correct] -> Switch3/2
  [conv] -> csc_sqt_sequential_trigger/4
  csc_tup_time_update/4 -> [conv]
  Bus Selector1/5 -> csc_tup_time_update/6  "<convergence>"
  cfe_time_msg/1 -> [time]
  csu_mkf_multiplicative_update_new/2 -> telem_bus/1
  [landed] -> csu_mkf_multiplicative_update_new/4
  [landed] -> csc_tup_time_update/4
  Bus Selector1/4 -> [landed], Logical Operator3/1  "<landed>"
  [time] -> csc_tup_time_update/8
  [q_ref] -> csc_tup_time_update/2
  Bus Selector1/3 -> csc_tup_time_update/3  "<P>"
  csu_mkf_multiplicative_update_new/1 -> new_state_bus/1
  sensor_bus/1 -> Bus Selector2/1, csu_mkf_multiplicative_update_new/6, csc_sqt_sequential_trigger/5, csc_tup_time_update/7
  Bus Selector1/1 -> csc_tup_time_update/1  "<x>"
  old_state_bus/1 -> Bus Selector1/1
  Bus Selector1/2 -> [q_ref]  "<q>"
  [q_ref] -> csu_mkf_multiplicative_update_new/2
  csc_tup_time_update/1 -> [xhat]
  [xhat] -> csc_sqt_sequential_trigger/1
  csc_tup_time_update/2 -> [qhat]
  [qhat] -> csc_sqt_sequential_trigger/2
  csc_tup_time_update/3 -> [P]
  [P] -> csc_sqt_sequential_trigger/3
  csc_sqt_sequential_trigger/1 -> Switch1/1
  [xhat] -> Switch1/3
  csc_sqt_sequential_trigger/2 -> Switch2/1
  Bus Selector2/1 -> Sum of Elements/1  "<meas_index>"
  Sum of Elements/1 -> Compare To Constant/1
  [correct] -> Switch1/2
  [P] -> Switch2/3
  [correct] -> Switch2/2
  Switch1/1 -> csu_mkf_multiplicative_update_new/1
  [time] -> csc_sqt_sequential_trigger/6
  [time] -> csu_mkf_multiplicative_update_new/7
  Bus Selector3/1 -> [frame_cmd]  "<est_ref_frame>"
  cmp_bus_msg/1 -> Bus Selector3/1
  [frame_cmd] -> csc_tup_time_update/9
  [frame_cmd] -> csu_mkf_multiplicative_update_new/8

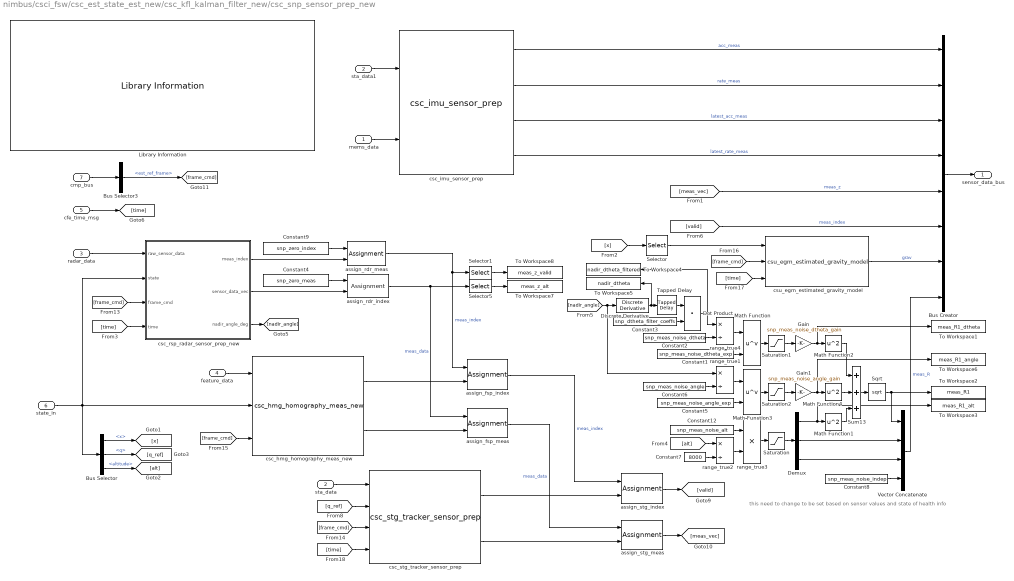
== system nimbus/csci_fsw/csc_est_state_est_new/csc_kfl_kalman_filter_new/csc_snp_sensor_prep_new ==
  note: this need to change to be set based on sensor values and state of health info
  mems_data : Inport
  sta_data : Inport  Port=2
  radar_data : Inport  Port=3
  feature_data : Inport  Port=4
  cfe_time_msg : Inport  Port=5
  state_in : Inport  Port=6
  cmp_bus : Inport  Port=7
  Bus Creator : BusCreator  Inputs=8
  Bus Selector : BusSelector  OutputSignals=x,q,altitude
  Bus Selector3 : BusSelector  OutputSignals=est_ref_frame
  Constant1 : Constant  Value=snp_meas_noise_dtheta_exp
  Constant12 : Constant  Value=snp_meas_noise_alt
  Constant2 : Constant  Value=snp_meas_noise_dtheta
  Constant3 : Constant  Value=snp_dtheta_filter_coeffs
  Constant4 : Constant  Value=snp_zero_meas
  Constant5 : Constant  Value=snp_meas_noise_angle_exp
  Constant6 : Constant  Value=snp_meas_noise_angle
  Constant7 : Constant  Value=8000
  Constant8 : Constant  Value=snp_meas_noise_indep
  Constant9 : Constant  Value=snp_zero_index
  Demux : Demux  Outputs=3
  Discrete Derivative : simulink/Discrete/Discrete Derivative  gainval=1.0  ICPrevScaledInput=0.0  InputProcessing=Inherited  OutMin=[]  OutMax=[]  OutDataType=fixdt(1, 16)  OutScaling=2^-10  DoSatur=off
  Dot Product : DotProduct  InputSameDT=on  OutDataTypeStr=Inherit: Inherit via internal rule
  Gain : Gain  Gain=snp_meas_noise_dtheta_gain
  Gain1 : Gain  Gain=snp_meas_noise_angle_gain
  Library Information : util_info_lib/Library Information  owner='NONE'
  Math Function : Math  Operator=pow  SaturateOnIntegerOverflow=on
  Math Function1 : Math  Operator=square  SaturateOnIntegerOverflow=on
  Math Function2 : Math  Operator=square  SaturateOnIntegerOverflow=on
  Math Function3 : Math  Operator=pow  SaturateOnIntegerOverflow=on
  Math Function4 : Math  Operator=square  SaturateOnIntegerOverflow=on
  Saturation : Saturate  UpperLimit=1e20*[1 1 1]  LowerLimit=snp_R_lower_limit_alt
  Saturation1 : Saturate  UpperLimit=1e20  LowerLimit=snp_R_lower_limit_dtheta
  Saturation2 : Saturate  UpperLimit=1e20  LowerLimit=snp_R_lower_limit_angle
  Selector : Selector  InputPortWidth=kfl_n_state  IndexOptions=Index vector (dialog)  Indices=kfl_pos_index  OutputSizes=1
  Selector1 : Selector  InputPortWidth=kfl_n_meas  IndexOptions=Index vector (dialog)  Indices=snp_rdr_index  OutputSizes=1
  Selector5 : Selector  InputPortWidth=kfl_n_meas  IndexOptions=Index vector (dialog)  Indices=snp_rdr_index  OutputSizes=1
  Sqrt : Sqrt  SaturateOnIntegerOverflow=on
  Sum13 : Sum  Inputs=+++
  Tapped Delay : simulink/Discrete/Tapped Delay  vinit=0.0  samptime=-1  NumDelays=snp_dtheta_filter_order  DelayOrder=Oldest  includeCurrent=on
  To Workspace1 : ToWorkspace  VariableName=meas_R1_dtheta  SaveFormat=Structure With Time  SampleTime=-1
  To Workspace2 : ToWorkspace  VariableName=meas_R1  SaveFormat=Structure With Time  SampleTime=-1
  To Workspace3 : ToWorkspace  VariableName=meas_R1_alt  SaveFormat=Structure With Time  SampleTime=-1
  To Workspace4 : ToWorkspace  VariableName=nadir_dtheta_filtered  SaveFormat=Structure With Time  SampleTime=-1
  To Workspace5 : ToWorkspace  VariableName=nadir_dtheta  SaveFormat=Structure With Time  SampleTime=-1
  To Workspace6 : ToWorkspace  VariableName=meas_R1_angle  SaveFormat=Structure With Time  SampleTime=-1
  To Workspace7 : ToWorkspace  VariableName=meas_z_alt  SaveFormat=Structure With Time  SampleTime=-1
  To Workspace8 : ToWorkspace  VariableName=meas_z_valid  SaveFormat=Structure With Time  SampleTime=-1
  Vector Concatenate : Concatenate  NumInputs=4
  assign_fsp_index : Assignment  IndexOptions=Index vector (dialog)  Indices=snp_fsp_index  OutputSizes=1
  assign_fsp_meas : Assignment  IndexOptions=Index vector (dialog)  Indices=snp_fsp_index  OutputSizes=1
  assign_rdr_index : Assignment  IndexOptions=Index vector (dialog)  Indices=snp_rdr_index  OutputSizes=1
  assign_rdr_meas : Assignment  IndexOptions=Index vector (dialog)  Indices=snp_rdr_index  OutputSizes=1
  assign_stg_index : Assignment  IndexOptions=Index vector (dialog)  Indices=snp_stg_index  OutputSizes=1
  assign_stg_meas : Assignment  IndexOptions=Index vector (dialog)  Indices=snp_stg_index  OutputSizes=1
  csc_hmg_homography_meas_new : csc_hmg_homoraphy_meas_lib/csc_hmg_homography_meas_new
  csc_imu_sensor_prep : csc_imu_sensor_prep_lib/csc_imu_sensor_prep
  csc_rsp_radar_sensor_prep_new : Subsystem  AncestorBlock=csc_rsp_radar_sensor_prep_lib/csc_rsp_radar_sensor_prep_new
  csc_stg_tracker_sensor_prep : csc_stg_tracker_sensor_prep_lib/csc_stg_tracker_sensor_prep
  csu_egm_estimated_gravity_model : csu_egm_estimated_gravity_model_lib/csu_egm_estimated_gravity_model
  range_true1 : Product  Inputs=*/  RndMeth=Zero
  range_true2 : Product  Inputs=*/  RndMeth=Zero
  range_true3 : Product  RndMeth=Zero
  range_true4 : Product  Inputs=*/  RndMeth=Zero
  sta_data1 : InportShadow  Port=2
  sensor_data_bus : Outport
  wires:
  [time] -> csc_stg_tracker_sensor_prep/4
  Constant8/1 -> Vector Concatenate/4
  Vector Concatenate/1 -> Bus Creator/8  "meas_R"
  Saturation/1 -> Demux/1
  Bus Selector3/1 -> [frame_cmd]  "<est_ref_frame>"
  [time] -> csu_egm_estimated_gravity_model/3
  [frame_cmd] -> csu_egm_estimated_gravity_model/2
  [frame_cmd] -> csc_hmg_homography_meas_new/3
  [frame_cmd] -> csc_stg_tracker_sensor_prep/3
  [frame_cmd] -> csc_rsp_radar_sensor_prep_new/3(frame_cmd)
  cmp_bus/1 -> Bus Selector3/1
  csc_stg_tracker_sensor_prep/1 -> assign_stg_index/2
  csc_stg_tracker_sensor_prep/2 -> assign_stg_meas/2
  assign_fsp_meas/1 -> assign_stg_meas/1  "meas_data"
  assign_stg_meas/1 -> [meas_vec]
  assign_stg_index/1 -> [valid]
  assign_fsp_index/1 -> assign_stg_index/1  "meas_index"
  [q_ref] -> csc_stg_tracker_sensor_prep/2
  Bus Selector/2 -> [q_ref]  "<q>"
  sta_data/1 -> csc_stg_tracker_sensor_prep/1
  Constant7/1 -> range_true2/2
  [alt] -> range_true2/1
  cfe_time_msg/1 -> [time]
  range_true3/1 -> Saturation/1
  Constant12/1 -> range_true3/1
  range_true2/1 -> range_true3/2
  Selector/1 -> csu_egm_estimated_gravity_model/1
  Bus Creator/1 -> sensor_data_bus/1
  csc_rsp_radar_sensor_prep_new/1(meas_index) -> assign_rdr_meas/2
  radar_data/1 -> csc_rsp_radar_sensor_prep_new/1(raw_sensor_data)
  [meas_vec] -> Bus Creator/5  "meas_z"
  csu_egm_estimated_gravity_model/1 -> Bus Creator/7  "grav"
  state_in/1 -> csc_rsp_radar_sensor_prep_new/2(state), csc_hmg_homography_meas_new/2, Bus Selector/1
  [x] -> Selector/1
  Bus Selector/1 -> [x]  "<x>"
  csc_hmg_homography_meas_new/2 -> assign_fsp_meas/2
  assign_rdr_index/1 -> assign_fsp_meas/1, Selector5/1  "meas_data"
  assign_rdr_meas/1 -> Selector1/1, assign_fsp_index/1  "meas_index"
  [valid] -> Bus Creator/6  "meas_index"
  feature_data/1 -> csc_hmg_homography_meas_new/1
  csc_rsp_radar_sensor_prep_new/2(sensor_data_vec) -> assign_rdr_index/2
  Constant4/1 -> assign_rdr_index/1
  Constant9/1 -> assign_rdr_meas/1
  csc_hmg_homography_meas_new/1 -> assign_fsp_index/2
  csc_imu_sensor_prep/1 -> Bus Creator/1  "acc_meas"
  csc_imu_sensor_prep/2 -> Bus Creator/2  "rate_meas"
  csc_imu_sensor_prep/3 -> Bus Creator/3  "latest_acc_meas"
  csc_imu_sensor_prep/4 -> Bus Creator/4  "latest_rate_meas"
  sta_data1/1 -> csc_imu_sensor_prep/1
  mems_data/1 -> csc_imu_sensor_prep/2
  [time] -> csc_rsp_radar_sensor_prep_new/4(time)
  Bus Selector/3 -> [alt]  "<altitude>"
  Demux/3 -> Vector Concatenate/3
  Demux/2 -> Vector Concatenate/2
  Demux/1 -> To Workspace3/1, Math Function1/1
  Saturation1/1 -> Gain/1
  Math Function/1 -> Saturation1/1
  range_true4/1 -> Math Function/1
  csc_rsp_radar_sensor_prep_new/3(nadir_angle_deg) -> [nadir_angle]
  Constant2/1 -> range_true4/2
  Dot Product/1 -> range_true4/1, To Workspace4/1
  Sum13/1 -> Sqrt/1
  Sqrt/1 -> Vector Concatenate/1, To Workspace2/1
  Math Function2/1 -> Sum13/1
  Math Function1/1 -> Sum13/3
  Tapped Delay/1 -> Dot Product/1
  Constant3/1 -> Dot Product/2
  Discrete Derivative/1 -> To Workspace5/1, Tapped Delay/1
  Saturation2/1 -> Gain1/1
  Math Function3/1 -> Saturation2/1
  range_true1/1 -> Math Function3/1
  Constant1/1 -> Math Function/2
  Constant6/1 -> range_true1/2
  [nadir_angle] -> range_true1/1, Discrete Derivative/1
  Math Function4/1 -> Sum13/2
  Gain/1 -> To Workspace1/1, Math Function2/1
  Gain1/1 -> To Workspace6/1, Math Function4/1
  Constant5/1 -> Math Function3/2
  Selector5/1 -> To Workspace7/1
  Selector1/1 -> To Workspace8/1

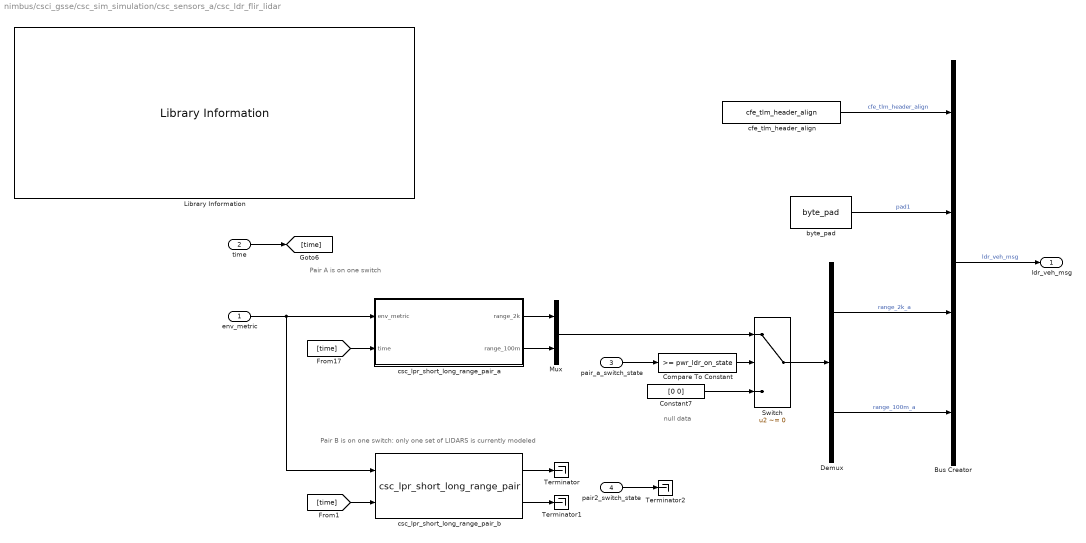
== system nimbus/csci_gsse/csc_sim_simulation/csc_sensors_a/csc_ldr_flir_lidar ==
  note: null data
  note: Pair A is on one switch
  note: Pair B is on one switch: only one set of LIDARS is currently modeled
  env_metric : Inport
  time : Inport  Port=2
  pair_a_switch_state : Inport  Port=3
  pair2_switch_state : Inport  Port=4
  Bus Creator : BusCreator  Inputs=4  OutDataTypeStr=Bus: ldr_veh_msg  NonVirtualBus=on
  Compare To Constant : simulink/Logic and Bit Operations/Compare To Constant  relop=>=  const=pwr_ldr_on_state  OutDataTypeStr=boolean
  Constant7 : Constant  Value=[0 0]  OutDataTypeStr=double
  Demux : Demux  Outputs=2
  Library Information : util_info_lib/Library Information  owner='escrane'
  Mux : Mux  Inputs=2
  Switch : Switch  Criteria=u2 ~= 0
  Terminator : Terminator
  Terminator1 : Terminator
  Terminator2 : Terminator
  byte_pad : util_common_lib/byte_pad  n_bytes=4
  cfe_tlm_header_align : util_common_lib/cfe_tlm_header_align
  csc_lpr_short_long_range_pair_a : Subsystem  AncestorBlock=csc_lpr_lidar_short_long_range_pair_lib/csc_lpr_short_long_range_pair  SystemSampleTime=0.1
  csc_lpr_short_long_range_pair_b : csc_lpr_lidar_short_long_range_pair_lib/csc_lpr_short_long_range_pair
  ldr_veh_msg : Outport
  wires:
  Bus Creator/1 -> ldr_veh_msg/1  "ldr_veh_msg"
  Demux/1 -> Bus Creator/3  "range_2k_a"
  env_metric/1 -> csc_lpr_short_long_range_pair_b/1, csc_lpr_short_long_range_pair_a/1(env_metric)
  Demux/2 -> Bus Creator/4  "range_100m_a"
  [time] -> csc_lpr_short_long_range_pair_a/2(time)
  time/1 -> [time]
  byte_pad/1 -> Bus Creator/2  "pad1"
  cfe_tlm_header_align/1 -> Bus Creator/1  "cfe_tlm_header_align"
  [time] -> csc_lpr_short_long_range_pair_b/2
  csc_lpr_short_long_range_pair_b/1 -> Terminator/1
  csc_lpr_short_long_range_pair_b/2 -> Terminator1/1
  csc_lpr_short_long_range_pair_a/1(range_2k) -> Mux/1
  csc_lpr_short_long_range_pair_a/2(range_100m) -> Mux/2
  Mux/1 -> Switch/1
  Switch/1 -> Demux/1
  Compare To Constant/1 -> Switch/2
  pair_a_switch_state/1 -> Compare To Constant/1
  Constant7/1 -> Switch/3
  pair2_switch_state/1 -> Terminator2/1
